simulink model "attitude_rate_control_C4"  (R2016a)
settings: Solver=VariableStepAuto  StartTime=0.0  StopTime=10.0  RelTol=1e-3
undefined symbols (not defined in the file): I, tau_omega
settings Model: Creator=mgreiff  LastModifiedBy=mgreiff

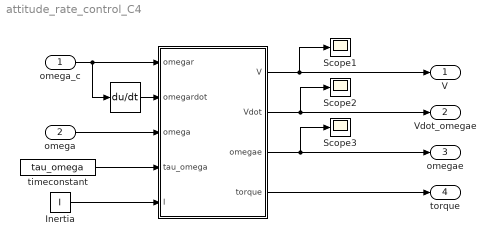
== system attitude_rate_control_C4 ==
  omega_c : Inport  PortDimensions=3
  omega : Inport  Port=2  PortDimensions=3
  " " : Derivative
  "     " : MATLAB Function  TreatAsAtomicUnit=on
  Inertia : Constant  Value=I
  Scope1 : Scope
  Scope2 : Scope
  Scope3 : Scope
  timeconstant : Constant  Value=tau_omega
  V : Outport  PortDimensions=1
  Vdot_omegae : Outport  Port=2  PortDimensions=1
  omegae : Outport  Port=3  PortDimensions=3
  torque : Outport  Port=4  PortDimensions=3
  wires:
  omega_c/1 -> " "/1, "     "/1(omegar)
  "     "/4(torque) -> torque/1
  timeconstant/1 -> "     "/4(tau_omega)
  "     "/1(V) -> V/1, Scope1/1
  omega/1 -> "     "/3(omega)
  Inertia/1 -> "     "/5(I)
  " "/1 -> "     "/2(omegardot)
  "     "/3(omegae) -> omegae/1, Scope3/1
  "     "/2(Vdot) -> Vdot_omegae/1, Scope2/1

== matlab function attitude_rate_control_C4/      ==
  data: V output; Vdot output; omegae output; omegar input; omegardot input; omega input; torque output; tau_omega input; I input
function [V, Vdot, omegae, torque] = C4(omegar, omegardot, omega, tau_omega, I)
    % ~~~~~~~~~ Copyright (c) 2018 Marcus Greiff (see LICENCE.md) ~~~~~~~~~
    %
    % A feedback linearizing and exponentially stabilizing feedback law in
    % for the attitude rate dynamics of the cascade, at location (C4).
    %
    %    [V, Vdot, omegae, torque] = C4(omegar, omegardot, omega, tau_omega, I)
    %
    % The controller takes a reference rate "omegar" and its derivative 
    % (here computed numerically) as "omegardot". Furthermore, it takes a
    % measurement attitude rate "omega" and a timeconstant "tau_omega"
    % determining the pseed of the controller. The only parametrization
    % required to operate the controller is the inertial tensor I.
    %
    % The outputs are the lyapunov function in time, "V", its time
    % derivative "Vdot" the computed attitude rate error "omegae" and the
    % control signals used to drive the attitude rate dynamics of the
    % cascaded system, in "torque".
    omegae = (omegar - omega);
    torque = +(1/tau_omega).*I*omegae...
             + skew(omega)*(I*omega) + I*omegardot;
    
    V = (1/2).*omegae'*omegae;
    Vdot = -omegae'*omegae;
end

function S = skew(v)
    vx = v(1);
    vy = v(2);
    vz = v(3);
    S = [0 -vz vy; vz 0 -vx; -vy vx 0];
end
